simulink model "robosim1"  (Simulink 8.7)
settings: Solver=ode45  StartTime=0.0  StopTime=60  MaxStep=0.01  RelTol=1e-6
values from neighbouring files (symbols this model uses):
  Kd = dlqr(Amd, Bmd,eye(3),0.7)    [gazebo_parameters.m]    (also in gpc.m = dlqr(A, B, eye(3),1); kalman_filter.m; questao1.m = dlqr(Ad,Bd,Q,R); questao2.m = [-K,zeros(1,2);zeros(1,2) -K])
libraries: simulink x1
settings Model: Creator=DH55PJ02  LastModifiedBy=Regner
settings DataIOCC: SignalLoggingSaveFormat=ModelDataLogs
settings OptimizationCC: ExpressionDepthLimit=2147483647
settings DebuggingCC: SaveWithParameterizedLinksMsg=none  SignalResolutionControl=TryResolveAllWithWarning  MultiTaskCondExecSysMsg=none  FcnCallInpInsideContextMsg=UseLocalSettings  StateNameClashWarn=warning
settings HardwareCC: TargetUnknown=on
settings GRTTargetCC: TargetFcnLib=ansi_tfl_tmw.mat  CombineOutputUpdateFcns=off  GRTInterface=on

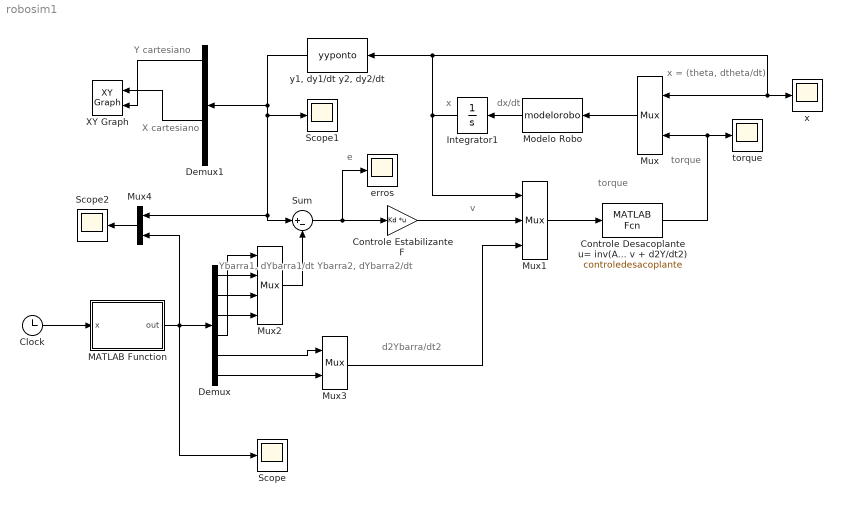
== system robosim1 ==
  note: x
  note: dx/dt
  note: torque
  note: Ybarra1, dYbarra1/dt
      |                               Ybarra2, dYbarra2/dt
  note: v
  note: d2Ybarra/dt2
  note: e
  note: torque
  note: x = (theta, dtheta/dt)
  note: Y cartesiano
  note: X cartesiano
  Clock : Clock
  Controle Desacoplante u= inv(A) (-a + v + d2Y/dt2) : MATLABFcn  MATLABFcn=controledesacoplante  OutputDimensions=2
  Controle Estabilizante F : Gain  Gain=Kd  Multiplication=Matrix(K*u)
  Demux : Demux  Outputs=6
  Demux1 : Demux
  Integrator1 : Integrator  InitialCondition=[0 pi/180*45 0 0]
  MATLAB Function : MATLAB Function  TreatAsAtomicUnit=on
  Modelo Robo : MATLABFcn  MATLABFcn=modelorobo  OutputDimensions=4
  Mux : Mux  Inputs=2
  Mux1 : Mux  Inputs=3
  Mux2 : Mux
  Mux3 : Mux  Inputs=2
  Mux4 : Mux  Inputs=2
  Scope : Scope
  Scope1 : Scope
  Scope2 : Scope
  Sum : Sum  Inputs=|+-
  XY Graph : simulink/Sinks/XY Graph  xmin=-2  xmax=2  ymin=-2  ymax=2  st=-1
  erros : Scope
  torque : Scope
  x : Scope
  "y1, dy1/dt y2, dy2/dt" : MATLABFcn  MATLABFcn=yyponto  OutputDimensions=4
  wires:
  Modelo Robo/1 -> Integrator1/1
  Mux/1 -> Modelo Robo/1
  Integrator1/1 -> "y1, dy1/dt y2, dy2/dt"/1, Mux/1, x/1, Mux1/1
  Controle Desacoplante u= inv(A) (-a + v + d2Y/dt2)/1 -> torque/1, Mux/2
  MATLAB Function/1(out) -> Scope/1, Mux4/2, Demux/1
  Mux1/1 -> Controle Desacoplante u= inv(A) (-a + v + d2Y/dt2)/1
  Sum/1 -> Controle Estabilizante F/1, erros/1
  Clock/1 -> MATLAB Function/1(x)
  Demux/1 -> Mux2/1
  Demux/2 -> Mux2/2
  Demux/3 -> Mux2/3
  Demux/4 -> Mux2/4
  Mux2/1 -> Sum/2
  Demux/5 -> Mux3/1
  Demux/6 -> Mux3/2
  Controle Estabilizante F/1 -> Mux1/2
  Mux3/1 -> Mux1/3
  Demux1/3 -> XY Graph/1
  Demux1/1 -> XY Graph/2
  "y1, dy1/dt y2, dy2/dt"/1 -> Scope1/1, Mux4/1, Sum/1, Demux1/1
  Mux4/1 -> Scope2/1

== matlab function MATLAB Function ==
  data: x input double; out output double
function out  = geracao(x)
t = x;
A = 0;
C = 1;
B = 1;
D = 1;
E = 1;
alfa = 2;
beta = 2;

if( 19<t)&&(t< 29)
    B = -1;
    C = 1;
end
if(29<t)&&(t< 39)
    B = -1;
    C = -1;
end
if(39<t)&&(t< 45)
    B = 1;
    C= -1;
end
if(49<t)&&(t<60)
    A = 1;
    B = 0;
    C = 0;
end
% yr1 = A*sin(t)+C;
% yr2 = A*cos(t)+B;
% 
% dyr1 = A*cos(t);
% dyr2 = -A*sin(t);
% 
% ddyr1 = -A*sin(t);
% ddyr2 = -A*cos(t);

yr1 = A*sin(t)+D*(1-exp(-alfa)*t)+C;
yr2 = A*cos(t)+E*(1-exp(-beta)*t)+B;

dyr1 = diff(yr1,t)
dyr2 = diff(yr2,t);

ddyr1 = diff(dyr1,t)
ddyr2 = diff(dyr2,t);

out = [yr1; dyr1; yr2; dyr2; ddyr1; ddyr2];
